simulink model "SIRV"  (R2023b)
settings: Solver=VariableStepAuto  StartTime=0.0  StopTime=10.0  RelTol=1e-3
model workspace (MAT data in the model file):
  I_0 = 0
  R_0 = 0
  S_0 = 1
  V_0 = 0
settings Model: Creator=simon  LastModifiedBy=simon

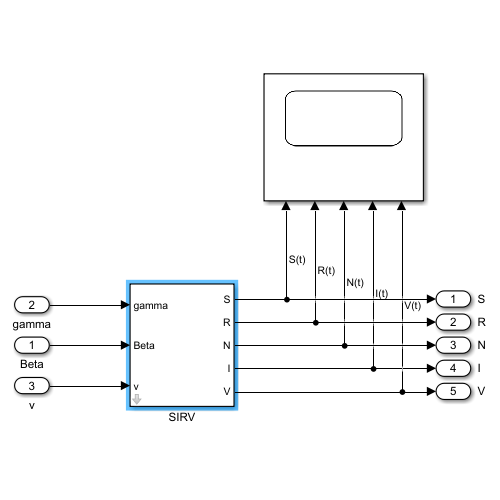
[thumbnail: Simulink's stored preview of the top-level diagram]
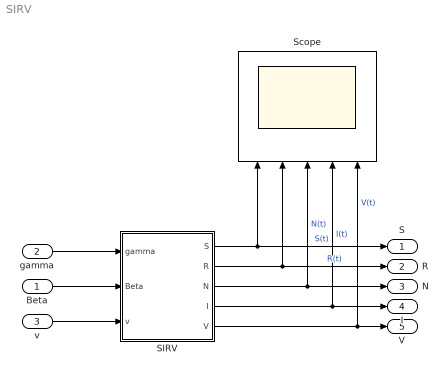
== system SIRV ==
  Beta : Inport
  gamma : Inport  Port=2
  v : Inport  Port=3
  SIRV : Subsystem  mask{B=1e-4, p=0.25, d=1e-4, Beta_0=0.2, gamma_0=0.1, nu_0=0, S_0=(1-1e-4), I_0=1e-4, R_0=0, V_0=0}
      mask prompts: B "Tasa de nacimientos"; p "Prob vacunacion natal"; d "Tasa de mortalidad natural"; Beta_0 "Tasa de Contactos Efectivos"; gamma_0 "Tasa de recuperacion"; nu_0 "Tasa de inmunizacion"; S_0 "Poblacion suceptible inicial"; I_0 "Poblacion infecciosos inicial"; R_0 "Poblacion recuperada inicial"; V_0 "Poblacion vacunada inicial"
  Scope : Scope  NumInputPorts=5
  S : Outport
  R : Outport  Port=2
  N : Outport  Port=3
  I : Outport  Port=4
  V : Outport  Port=5
  wires:
  gamma/1 -> SIRV/1(gamma)
  Beta/1 -> SIRV/2(Beta)
  v/1 -> SIRV/3(v)
  SIRV/1(S) -> S/1, Scope/1  "S(t)"
  SIRV/2(R) -> R/1, Scope/2  "R(t)"
  SIRV/3(N) -> N/1, Scope/3  "N(t)"
  SIRV/4(I) -> I/1, Scope/4  "I(t)"
  SIRV/5(V) -> V/1, Scope/5  "V(t)"

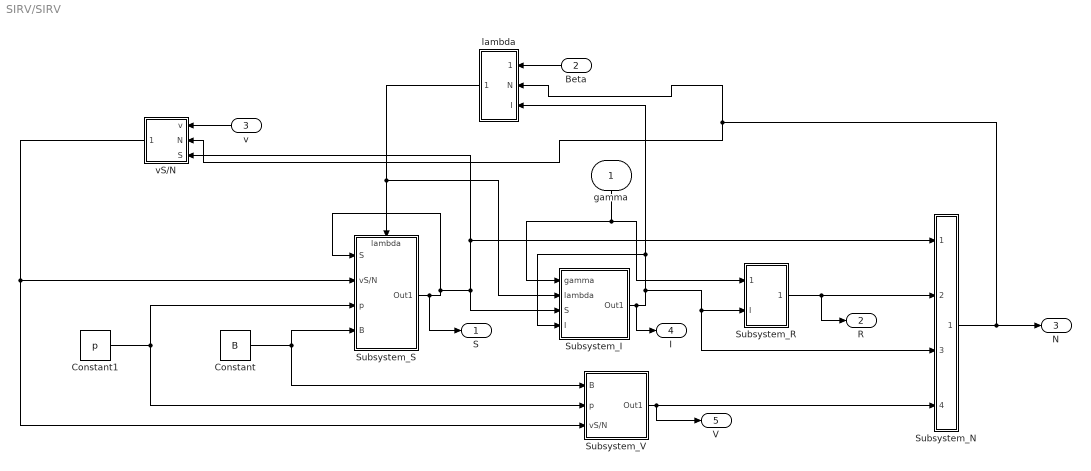
== system SIRV/SIRV ==
  gamma : Inport
  Beta : Inport  Port=2
  v : Inport  Port=3
  Constant : Constant  Value=B
  Constant1 : Constant  Value=p
  Subsystem_I : Subsystem
  Subsystem_N : Subsystem
  Subsystem_R : Subsystem
  Subsystem_S : Subsystem
      settings: PortSchema="{\"entries\":[{\"content\":{\"sides\":[{\"content\":{\"connectorIds\":[\"In1\",\"In2\",\"In3\",\"In4\"]},\"type\":\"ConnectorPlacement.EquallySpacedRectSide\",\"uuid\":\"66979525-184f-41f5-b5c9-003b2347c688\"},{\"content\":{\"connectorIds\":[\"Out1\"],\"side\":\"RIGHT\"},\"type\":\"ConnectorPlacement.EquallySpacedRectSide\",\"uuid\":\"c8d1f39b-cc4c-44b2-badf-e76855629269\"},{\"content\":{\"connectorIds\":[\"In5\"],\"side\":\"TOP\"},\"type\":\"ConnectorPlacement.EquallySpacedRectSide\",\"uuid\":\"58eb6ea7-df11-4795-94ba-341cf865bd24\"}]},\"type\":\"ConnectorPlacement.EquallySpacedConnector\",\"uuid\":\"253c02f8-130c-4a17-bf21-fe770be5f111\"}],\"packageUris\":[\"http://schema.mathworks.com/mf0/Connector/R2020b\"],\"version\":\"1.0\"}"
  Subsystem_V : Subsystem
  lambda : Subsystem
  vS/N : Subsystem
  S : Outport
  R : Outport  Port=2
  N : Outport  Port=3
  I : Outport  Port=4
  V : Outport  Port=5
  wires:
  Constant1/1 -> Subsystem_V/2(p), Subsystem_S/3(p)
  Subsystem_S/1(Out1) -> S/1, vS/N/3(S), Subsystem_N/1(S), Subsystem_I/3(S), Subsystem_S/1(S)
  vS/N/1(vS/N) -> Subsystem_V/3(vS/N), Subsystem_S/2(vS/N)
  lambda/1(lambda) -> Subsystem_I/2(lambda), Subsystem_S/5(lambda)
  Constant/1 -> Subsystem_S/4(B), Subsystem_V/1(B)
  Subsystem_N/1(Out1) -> N/1, vS/N/2(N), lambda/2(N)
  gamma/1 -> Subsystem_R/1(gamma), Subsystem_I/1(gamma)
  Subsystem_I/1(Out1) -> I/1, lambda/3(I), Subsystem_I/4(I), Subsystem_N/3(I), Subsystem_R/2(I)
  Subsystem_R/1(Out1) -> R/1, Subsystem_N/2(R)
  Subsystem_V/1(Out1) -> Subsystem_N/4(V), V/1
  v/1 -> vS/N/1(v)
  Beta/1 -> lambda/1(Beta)

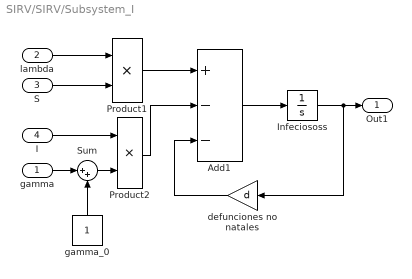
== system SIRV/SIRV/Subsystem_I ==
  gamma : Inport
  lambda : Inport  Port=2
  S : Inport  Port=3
  I : Inport  Port=4
  Add1 : Sum  Inputs=+--
  Infeciososs : Integrator  InitialCondition=I_0
  Product1 : Product
  Product2 : Product
  Sum : Sum  Inputs=|++
  defunciones no natales : Gain  Gain=d
  gamma_0 : Constant
  Out1 : Outport
  wires:
  defunciones no natales/1 -> Add1/3
  S/1 -> Product1/2
  Infeciososs/1 -> Out1/1, defunciones no natales/1
  Product1/1 -> Add1/1
  I/1 -> Product2/1
  Product2/1 -> Add1/2
  Add1/1 -> Infeciososs/1
  lambda/1 -> Product1/1
  gamma/1 -> Sum/1
  Sum/1 -> Product2/2
  gamma_0/1 -> Sum/2

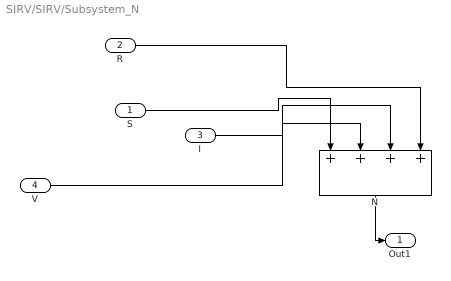
== system SIRV/SIRV/Subsystem_N ==
  S : Inport
  R : Inport  Port=2
  I : Inport  Port=3
  V : Inport  Port=4
  N : Sum  Inputs=++++
  Out1 : Outport
  wires:
  R/1 -> N/4
  N/1 -> Out1/1
  I/1 -> N/3
  S/1 -> N/1
  V/1 -> N/2

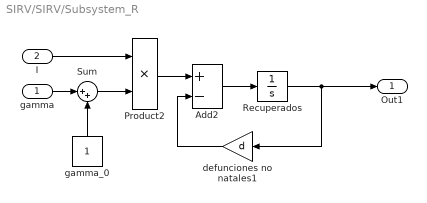
== system SIRV/SIRV/Subsystem_R ==
  gamma : Inport
  I : Inport  Port=2
  Add2 : Sum  Inputs=+-
  Product2 : Product
  Recuperados : Integrator  InitialCondition=R_0
  Sum : Sum  Inputs=|++
  defunciones no natales1 : Gain  Gain=d
  gamma_0 : Constant
  Out1 : Outport
  wires:
  Add2/1 -> Recuperados/1
  Recuperados/1 -> defunciones no natales1/1, Out1/1
  defunciones no natales1/1 -> Add2/2
  Product2/1 -> Add2/1
  I/1 -> Product2/1
  gamma/1 -> Sum/1
  gamma_0/1 -> Sum/2
  Sum/1 -> Product2/2

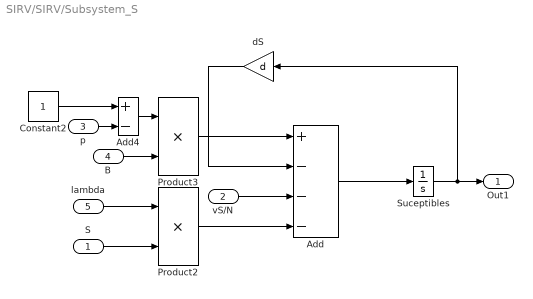
== system SIRV/SIRV/Subsystem_S ==
  S : Inport
  vS/N : Inport  Port=2
  p : Inport  Port=3
  B : Inport  Port=4
  lambda : Inport  Port=5
  Add : Sum  Inputs=+---
  Add4 : Sum  Inputs=+-
  Constant2 : Constant
  Product2 : Product
  Product3 : Product
  Suceptibles : Integrator  InitialCondition=S_0
  dS : Gain  Gain=d
  Out1 : Outport
  wires:
  Constant2/1 -> Add4/1
  Add/1 -> Suceptibles/1
  Suceptibles/1 -> Out1/1, dS/1
  Product2/1 -> Add/4
  lambda/1 -> Product2/1
  Add4/1 -> Product3/1
  Product3/1 -> Add/1
  dS/1 -> Add/2
  S/1 -> Product2/2
  vS/N/1 -> Add/3
  B/1 -> Product3/2
  p/1 -> Add4/2

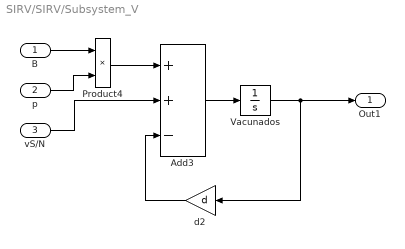
== system SIRV/SIRV/Subsystem_V ==
  B : Inport
  p : Inport  Port=2
  vS/N : Inport  Port=3
  Add3 : Sum  Inputs=++-
  Product4 : Product
  Vacunados : Integrator  InitialCondition=V_0
  d2 : Gain  Gain=d
  Out1 : Outport
  wires:
  d2/1 -> Add3/3
  Product4/1 -> Add3/1
  B/1 -> Product4/1
  Add3/1 -> Vacunados/1
  Vacunados/1 -> Out1/1, d2/1
  p/1 -> Product4/2
  vS/N/1 -> Add3/2

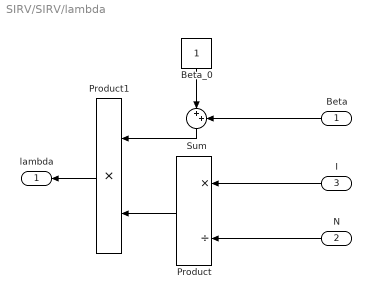
== system SIRV/SIRV/lambda ==
  Beta : Inport
  N : Inport  Port=2
  I : Inport  Port=3
  Beta_0 : Constant
  Product : Product  Inputs=*/
  Product1 : Product
  Sum : Sum  Inputs=|++
  lambda : Outport
  wires:
  N/1 -> Product/2
  Product/1 -> Product1/2
  I/1 -> Product/1
  Product1/1 -> lambda/1
  Sum/1 -> Product1/1
  Beta_0/1 -> Sum/1
  Beta/1 -> Sum/2

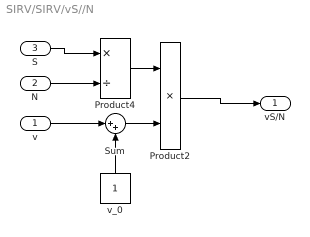
== system SIRV/SIRV/vS//N ==
  v : Inport
  N : Inport  Port=2
  S : Inport  Port=3
  Product2 : Product
  Product4 : Product  Inputs=*/
  Sum : Sum  Inputs=|++
  v_0 : Constant
  vS/N : Outport
  wires:
  S/1 -> Product4/1
  N/1 -> Product4/2
  v/1 -> Sum/1
  v_0/1 -> Sum/2
  Product2/1 -> vS/N/1
  Sum/1 -> Product2/2
  Product4/1 -> Product2/1
